simulink library "JT60SA_Magnetic_Control"  (R2019a)
settings: Solver=ode45  StartTime=0.0  StopTime=10.0  RelTol=1e-3  EnableMultiTasking=on
values from neighbouring files (symbols this model uses):
  Input_struct =     [SOF18d66_setup.mat]
  Ip0 = 5499999.99826    [SOF18d66_setup.mat]
  IVC_sat = 1000    [SOF18d66_setup.mat]
undefined symbols (not defined in the file or in its folder): iLow, Ip_PID, iUp, r_grid, R_grid, Rt, z_grid, Z_grid, Zt
libraries: simulink x2, cstblocks x2
settings Model: Creator=Adriano  LastModifiedBy=adria
settings DataIOCC: LimitDataPoints=on  SaveFormat=Array  ReturnWorkspaceOutputs=off
settings OptimizationCC: LifeSpan=inf
settings DebuggingCC: SFUnexpectedBacktrackingDiag=warning  SFNoUnconditionalDefaultTransitionDiag=warning  SFExecutionAtInitializationDiag=none  ArithmeticOperatorsInVariantConditions=warning
settings HardwareCC: ProdBitPerPointer=32  ProdBitPerSizeT=32  ProdBitPerPtrDiffT=32  ProdLargestAtomicFloat=None  ProdIntDivRoundTo=Undefined  ProdEndianess=Unspecified  ProdWordSize=32  ProdHWDeviceType=32-bit Generic
settings ModelReferenceCC: PropagateSignalLabelsOutOfModel=off
settings SFSimCC: SimUseLocalCustomCode=off
settings RTWCC: RTWUseLocalCustomCode=off
settings CodeAppCC: StateflowObjectComments=on
settings GRTTargetCC: TargetLangStandard=C89/C90 (ANSI)  GeneratePreprocessorConditionals=Disable all
settings ConfigComp: CovMetricSettings=dw  CovHtmlReporting=on  CovSaveCumulativeToWorkspaceVar=on  CovSaveSingleToWorkspaceVar=on  CovExternalEMLEnable=off

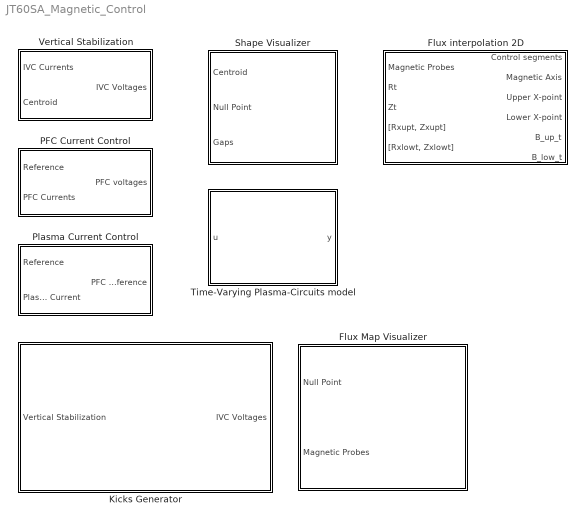
== system JT60SA_Magnetic_Control ==
  Flux Map Visualizer : Subsystem  InitFcn=|  StartFcn=% fig_grid= figure()
      | oldDir = pwd;
      | cd ./flux_grid_functions
      | [r_grid, z_grid, R_grid, Z_grid, F0, idxGrid] = initFluxGrid(Input_struct,y_np,y_type, mag, 0);
      | cd(oldDir);
      mask Display:
      | image(['.' filesep 'images' filesep 'Grid.jpg'])
      | port_label('input',1,'Null Point');
      | port_label('input',2, 'Mag Probes');
  Flux interpolation 2D : Subsystem  Description=|  InitFcn=|
      Description=|
      | This block allows to interpolate the flux map over a set of given control points.
      | 
      | The user must define Rt and Zt, which are 2 vectors of 20 elements which contain the coordinates
      | of the desired control points (only non-zero coordinate are used). Furthermore, the user must
      | define the desired position for the upper and lower X-points, [Rxupt, Zxupt] and [Rxlowt, Zxlowt]. 
      | The target points may be time varying.
      InitFcn=|
      | oldDir = pwd;
      | cd ./flux_grid_functions
      | [r_grid, z_grid, R_grid, Z_grid, F0, idxGrid] = initFluxGrid(Input_struct,y_np,y_type, mag, 0);
      | 
      | xpLow_guess = [Null0(1) -abs(Null0(2))];
      | [RBoxL, ZBoxL, irowL, icolL, maskL] = initXBox(xpLow_guess, R_grid, Z_grid);
      | iLow = [irowL; icolL];
      | 
      | xpUp_guess = [Null0(1) +abs(Null0(2))];
      | [RBoxU, ZBoxU, irowU, icolU, maskU] = initXBox(xpUp_guess, R_grid, Z_grid);
      | iUp = [irowU; icolU];
      | 
      | cd(oldDir);
  Kicks Generator : Subsystem  mask{freq_kicks=5, duty_cycle=50, perc_up=45}
      mask prompts: freq_kicks "Frequence [Hz]"; duty_cycle "Duty cycle"; perc_up "%up"
      mask Display:
      | image(['.' filesep 'images' filesep 'Kicks.png']);
      | port_label('input',1,'Vertical Stabilization');
      | port_label('output',1,'IVC Voltages');
  PFC Current Control : Subsystem  InitFcn=|
      | % PFC Current Control
      | Kpcurr = [5.7832    1.2410     0           0           0            0          0.8592   0            0            0
      |                1.2410    5.7862    1.2432    0           0            0          0           0            0            0
      |                0            1.2432    5.7865    1.2414   0            0          0           0            0            0
      |                0            0            1.2414    5.7845   0            0          0           0            0            0
      |                0            0            0            0           10.9807  2.7576  0           0            0.8679    2.0055
      |                0            0            0            0           2.7576    9.5196  1.2014   0            0            0
      |                0.8592    0            0            0           0            1.2014  6.6407   0            0            0
      |                0            0            0            1.1486   0            0          0           12.5627  2.1557    1.7044
      |                0            0            0            0           0            0          0           2.1557    7.4827    3.7590
      |                0            0            0            0           2.0055    0          0           1.7044    3.7590   14.2743]; % Decoupling Matrix
      mask help: PF Coils Current Controller
      mask init:
      | Kpcurr = [5.7832   1.2410        0        0         0       0  0.8592        0        0         0
      |           1.2410   5.7862   1.2432        0         0       0       0        0        0         0
      |                0   1.2432   5.7865   1.2414         0       0       0        0        0         0
      |                0        0   1.2414   5.7845         0       0       0        0        0         0
      |                0        0        0        0   10.9807  2.7576       0        0   0.8679    2.0055
      |                0        0        0        0    2.7576  9.5196  1.2014        0        0         0
      |           0.8592        0        0        0         0  1.2014  6.6407        0        0         0
      |                0        0        0   1.1486         0       0       0  12.5627   2.1557    1.7044
      |                0        0        0        0         0       0       0   2.1557   7.4827    3.7590
      |                0        0        0        0    2.0055       0       0   1.7044   3.7590   14.2743];
  Plasma Current Control : Subsystem  InitFcn=|  mask{Ip_Kp=1e-3, Ip_Ki=35*1e-3}
      | % Ip Control
      |  KIp= [-0.4984  -0.4327  -0.4393 -0.4969  -0.0241 ...
      |         -0.0268  -0.2920  -0.1886  -0.0465  -0.0151]'; % Transformer currents pattern
      mask prompts: Ip_Kp "Proportional gain"; Ip_Ki "Integral gain"
      mask help: Plasma Current Controller
      mask init:
      | KIp= [-0.4984  -0.4327  -0.4393 -0.4969  -0.0241 ...
      |       -0.0268  -0.2920  -0.1886  -0.0465 -0.0151]'; % Transformer currents pattern, normalized
  Shape Visualizer : Subsystem  StartFcn=|
      | plasmaShape = figure('Position',[800, 0, 450, 650]);
      | xlabel('R');
      | ylabel('Z');
      | 
      | %h = pdemesh(Input_struct.p,Input_struct.e,[]);
      | %set(h,'Color','black');
      | %axis([0, 6, -4.5, 4.5]);
      | %axis equal;
      | %hold on
      | 
      | %plasmaShape.UserData.plot = plot(zeros(nGaps,1), zeros(nGaps,1));
      mask help: Plasma Shape Visualizer
      mask Display:
      | image(['.' filesep 'images' filesep 'Shape.JPG']);
      | port_label('input',1,'Centroid');
      | port_label('input',2, 'Null Point');
      | port_label('input',3, 'Gaps');
  Time-Varying Plasma-Circuits model : Subsystem  InitFcn=|
      | if ~exist('equ_struct', 'var')
      |   try
      |       firstEquil = [pathName, fileName];
      |   catch
      |   end
      | 
      |   addpath(['.' filesep 'time-varying_model'])
      |   gen_equil_struct;
      | 
      | else
      |   warndlg('Equilibria structure already exists!');
      | end
      mask help: Time-Varying Plasma-Circuits linearized model.
      settings: DeleteFcn=clear equ_struct
      settings: CopyFcn=|
      | if ~exist('equ_struct', 'var')
      |   try
      |       firstEquil = [pathName, fileName];
      |   catch
      |   end
      | 
      |   addpath(['.' filesep 'time-varying_model'])
      |   gen_equil_struct;
      | else
      |   warndlg('Equilibria structure already exists!')
      | end
      mask Help:
      | This block contains a Time-Varying Plasma-Circuits model.
      | At the initialization, the user is asked to choose the equilibria to load
      | (the first one is the one currently loaded in the workspace). After this,
      | the user is asked to specify a time vector (one time istant for each model).
      | This block can be substituted to the blocks CREATE Model, Equilibrium
      | Inputs and Equilibrium Outputs under the Plasma-Circuits Linearized Model
      | mask (please note that the equilibrium inputs and outputs are already
      | taken into account, so the must not be added externally).
      | 
      | In the workspace, a structure named equ_struct will be available,
      | containing, among the other fields, the scenario currents for each of the
      | equilibria (these can be interpolated to build the current feedforward to
      | the model).
  Vertical Stabilization : Subsystem  InitFcn=|  mask{Zdot_Gain=-20/5.5e6, IVC_Gain=0.0076, VS_Gain=40}
      | % Vertical Stabilization
      | Zdot_Gain = 20;
      | IVC_Gain  = -0.0076;
      | VS_Gain   = -40;
      | derivativeFilter = tf([1, 0], [1/1000, 1]);
      mask prompts: Zdot_Gain "Velocity Gain/Ip"; IVC_Gain "Current Gain"; VS_Gain "Overall Gain"
      mask help: Vertical Stabilization Controller
      mask init:
      | % Zdot_Gain = 20/5.5e6;
      | % IVC_Gain  = -0.0076;
      | % VS_Gain   = -40;
      | 
      | derivativeFilter = tf([1, 0], [1/1000, 1]);

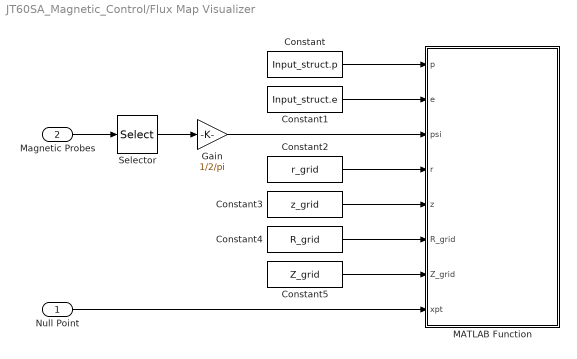
== system JT60SA_Magnetic_Control/Flux Map Visualizer ==
  Null Point : Inport
  Magnetic Probes : Inport  Port=2
  Constant : Constant  Value=Input_struct.p
  Constant1 : Constant  Value=Input_struct.e
  Constant2 : Constant  Value=r_grid
  Constant3 : Constant  Value=z_grid
  Constant4 : Constant  Value=R_grid
  Constant5 : Constant  Value=Z_grid
  Gain : Gain  Gain=1/2/pi
  MATLAB Function : MATLAB Function  TreatAsAtomicUnit=on  SystemSampleTime=5e-2
  Selector : Selector  InputPortWidth=nMag  IndexOptions=Index vector (dialog)  Indices=idxGrid  OutputSizes=1
  wires:
  Magnetic Probes/1 -> Selector/1
  Selector/1 -> Gain/1
  Constant/1 -> MATLAB Function/1(p)
  Constant1/1 -> MATLAB Function/2(e)
  Constant2/1 -> MATLAB Function/4(r)
  Constant3/1 -> MATLAB Function/5(z)
  Constant4/1 -> MATLAB Function/6(R_grid)
  Constant5/1 -> MATLAB Function/7(Z_grid)
  Null Point/1 -> MATLAB Function/8(xpt)
  Gain/1 -> MATLAB Function/3(psi)

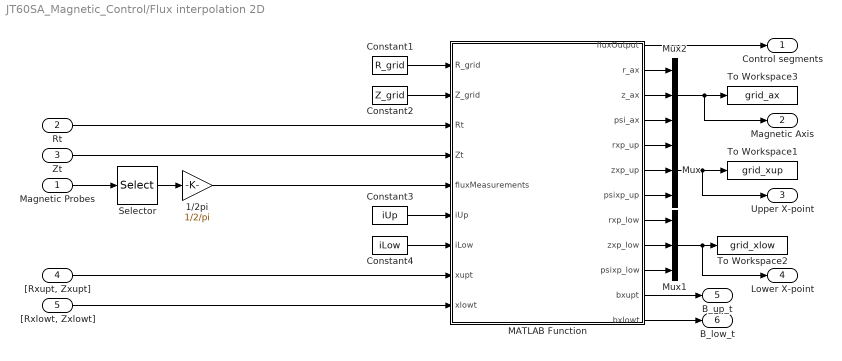
== system JT60SA_Magnetic_Control/Flux interpolation 2D ==
  Magnetic Probes : Inport
  Rt : Inport  Port=2
  Zt : Inport  Port=3
  "[Rxupt, Zxupt]" : Inport  Port=4
  "[Rxlowt, Zxlowt]" : Inport  Port=5
  1/2pi : Gain  Gain=1/2/pi
  Constant1 : Constant  Value=R_grid
  Constant2 : Constant  Value=Z_grid
  Constant3 : Constant  Value=iUp
  Constant4 : Constant  Value=iLow
  MATLAB Function : MATLAB Function  TreatAsAtomicUnit=on
  Mux : Mux  Inputs=3
  Mux1 : Mux  Inputs=3
  Mux2 : Mux  Inputs=3
  Selector : Selector  InputPortWidth=nMag  IndexOptions=Index vector (dialog)  Indices=idxGrid  OutputSizes=1
  To Workspace1 : ToWorkspace  VariableName=grid_xup  SaveFormat=Structure With Time  SampleTime=-1
  To Workspace2 : ToWorkspace  VariableName=grid_xlow  SaveFormat=Structure With Time  SampleTime=-1
  To Workspace3 : ToWorkspace  VariableName=grid_ax  SaveFormat=Structure With Time  SampleTime=-1
  Control segments : Outport
  Magnetic Axis : Outport  Port=2
  Upper X-point : Outport  Port=3
  Lower X-point : Outport  Port=4
  B_up_t : Outport  Port=5
  B_low_t : Outport  Port=6
  wires:
  Rt/1 -> MATLAB Function/3(Rt)
  Constant1/1 -> MATLAB Function/1(R_grid)
  Constant2/1 -> MATLAB Function/2(Z_grid)
  MATLAB Function/1(fluxOutput) -> Control segments/1
  Selector/1 -> 1/2pi/1
  Zt/1 -> MATLAB Function/4(Zt)
  Constant3/1 -> MATLAB Function/6(iUp)
  Constant4/1 -> MATLAB Function/7(iLow)
  MATLAB Function/5(rxp_up) -> Mux/1
  MATLAB Function/7(psixp_up) -> Mux/3
  MATLAB Function/6(zxp_up) -> Mux/2
  Mux/1 -> Upper X-point/1, To Workspace1/1
  MATLAB Function/8(rxp_low) -> Mux1/1
  MATLAB Function/9(zxp_low) -> Mux1/2
  MATLAB Function/10(psixp_low) -> Mux1/3
  Mux1/1 -> Lower X-point/1, To Workspace2/1
  MATLAB Function/2(r_ax) -> Mux2/1
  MATLAB Function/3(z_ax) -> Mux2/2
  MATLAB Function/4(psi_ax) -> Mux2/3
  Mux2/1 -> Magnetic Axis/1, To Workspace3/1
  MATLAB Function/11(bxupt) -> B_up_t/1
  "[Rxupt, Zxupt]"/1 -> MATLAB Function/8(xupt)
  "[Rxlowt, Zxlowt]"/1 -> MATLAB Function/9(xlowt)
  MATLAB Function/12(bxlowt) -> B_low_t/1
  Magnetic Probes/1 -> Selector/1
  1/2pi/1 -> MATLAB Function/5(fluxMeasurements)

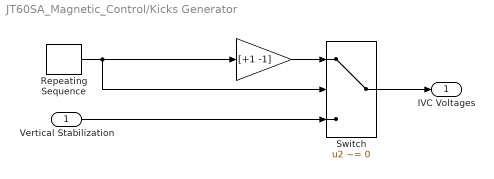
== system JT60SA_Magnetic_Control/Kicks Generator ==
  Vertical Stabilization : Inport
  "    " : Gain  Gain=[+1 -1]
  Repeating Sequence : simulink/Sources/Repeating Sequence  rep_seq_t="[0   (duty_cycle/100/freq_kicks)*(perc_up/100)+eps   (duty_cycle/100/freq_kicks)*(perc_up/100)+1.1*eps   duty_cycle/100/freq_kicks+1.2*eps  (duty_cycle/100/freq_kicks)+1.3*eps     1/freq_kicks+1.4*eps]"  rep_seq_y="[IVC_sat  IVC_sat   -IVC_sat  -IVC_sat  0  0]"
  Switch : Switch  Criteria=u2 ~= 0
  IVC Voltages : Outport
  wires:
  Switch/1 -> IVC Voltages/1
  "    "/1 -> Switch/1
  Repeating Sequence/1 -> "    "/1, Switch/2
  Vertical Stabilization/1 -> Switch/3

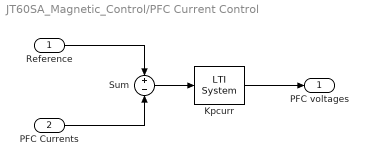
== system JT60SA_Magnetic_Control/PFC Current Control ==
  Reference : Inport
  PFC Currents : Inport  Port=2
  Kpcurr : cstblocks/LTI System  sys=Kpcurr  IC=[]
  Sum : Sum  Inputs=+-
  PFC voltages : Outport
  wires:
  Sum/1 -> Kpcurr/1
  PFC Currents/1 -> Sum/2
  Reference/1 -> Sum/1
  Kpcurr/1 -> PFC voltages/1

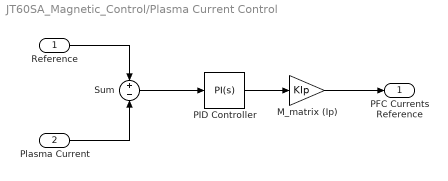
== system JT60SA_Magnetic_Control/Plasma Current Control ==
  Reference : Inport
  Plasma Current : Inport  Port=2
  M_matrix (Ip) : Gain  Gain=KIp
  PID Controller : simulink/Continuous/PID Controller  Controller=PI  Form=Parallel  TimeDomain=Continuous-time  SampleTime=-1  IntegratorMethod=Forward Euler  FilterMethod=Forward Euler  ControllerParametersSource=internal  P=Ip_Kp  I=Ip_Ki  D=Ip_PID.Kd  UseFilter=on  N=Ip_PID.Td  TunerSelectOption=Transfer Function Based (PID Tuner App)  InitialConditionSource=internal  InitialConditionForIntegrator=0  InitialConditionForFilter=0  DifferentiatorICPrevScaledInput=0  ExternalReset=none  TrackingMode=off  Kt=1  LimitOutput=off  UpperSaturationLimit=inf  LowerSaturationLimit=-inf  LinearizeAsGain=on  AntiWindupMode=none  Kb=1  POutMin=[]  POutMax=[]  IOutMin=[]  IOutMax=[]  DOutMin=[]  DOutMax=[]  NOutMin=[]  NOutMax=[]  SumOutMin=[]  SumOutMax=[]  SaturationOutMin=[]  SaturationOutMax=[]  PParamMin=[]  PParamMax=[]  IParamMin=[]  IParamMax=[]  DParamMin=[]  DParamMax=[]  NParamMin=[]  NParamMax=[]  KbParamMin=[]  KbParamMax=[]  KtParamMin=[]  KtParamMax=[]  KbOutMin=[]  KbOutMax=[]  KtOutMin=[]  KtOutMax=[]  IntegratorOutMin=[]  IntegratorOutMax=[]  FilterOutMin=[]  FilterOutMax=[]  SumI1OutMin=[]  SumI1OutMax=[]  SumI2OutMin=[]  SumI2OutMax=[]  SumI3OutMin=[]  SumI3OutMax=[]  SumI4OutMin=[]  SumI4OutMax=[]  SumDOutMin=[]  SumDOutMax=[]  DifferentiatorOutMin=[]  DifferentiatorOutMax=[]  FilterDiffOutCoefMin=[]  FilterDiffOutCoefMax=[]  ReciprocalOutMin=[]  ReciprocalOutMax=[]  SumDenOutMin=[]  SumDenOutMax=[]  SumNumOutMin=[]  SumNumOutMax=[]  DivideOutMin=[]  DivideOutMax=[]  IntegratorContinuousStateAttributes=''  IntegratorStateMustResolveToSignalObject=off  IntegratorRTWStateStorageClass=Auto  FilterContinuousStateAttributes=''  FilterStateMustResolveToSignalObject=off  FilterRTWStateStorageClass=Auto  ParallelPVariant=InternalParameters  IdealPVariant=Disabled  IVariant=InternalParameters  DVariant=Disabled  IntegratorVariant=Continuous  SatVariant=Disabled  AWVariant=Passthrough  PCopyVariant=Disabled  TRVariant=Disabled  FdbkBlocksVariant=Forward  IdealPFdbkVariant=Disabled  SatFdbkVariant=Disabled  DerivativeFilterVariant=Disabled  NVariant=Disabled  NCopyVariant=Disabled_SignalSpec  FilterICVariant=Disabled  IntegratorICVariant=InternalICs  ExternalResetVariant=Disabled  TRSumVariant=Passthrough  SumFdbkVariant=Disabled  SumVariant=Sum_PI
  Sum : Sum  Inputs=+-
  PFC Currents Reference : Outport
  wires:
  M_matrix (Ip)/1 -> PFC Currents Reference/1
  Sum/1 -> PID Controller/1
  PID Controller/1 -> M_matrix (Ip)/1
  Reference/1 -> Sum/1
  Plasma Current/1 -> Sum/2

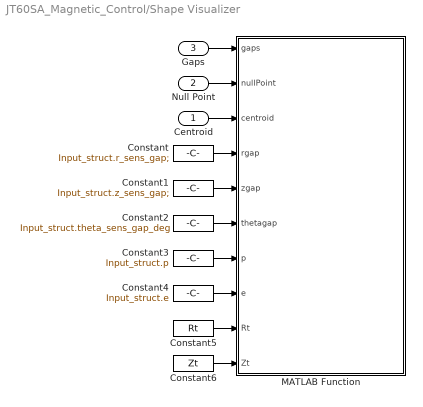
== system JT60SA_Magnetic_Control/Shape Visualizer ==
  Centroid : Inport  OutDataTypeStr=double  SampleTime=.05
  Null Point : Inport  Port=2  OutDataTypeStr=double  SampleTime=.05
  Gaps : Inport  Port=3  OutDataTypeStr=double  SampleTime=.05
  Constant : Constant  Value=Input_struct.r_sens_gap;
  Constant1 : Constant  Value=Input_struct.z_sens_gap;
  Constant2 : Constant  Value=Input_struct.theta_sens_gap_deg
  Constant3 : Constant  Value=Input_struct.p
  Constant4 : Constant  Value=Input_struct.e
  Constant5 : Constant  Value=Rt
  Constant6 : Constant  Value=Zt
  MATLAB Function : MATLAB Function  TreatAsAtomicUnit=on
  wires:
  Constant/1 -> MATLAB Function/4(rgap)
  Constant1/1 -> MATLAB Function/5(zgap)
  Constant2/1 -> MATLAB Function/6(thetagap)
  Gaps/1 -> MATLAB Function/1(gaps)
  Constant3/1 -> MATLAB Function/7(p)
  Constant4/1 -> MATLAB Function/8(e)
  Null Point/1 -> MATLAB Function/2(nullPoint)
  Centroid/1 -> MATLAB Function/3(centroid)
  Constant5/1 -> MATLAB Function/9(Rt)
  Constant6/1 -> MATLAB Function/10(Zt)

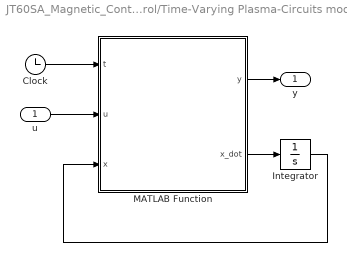
== system JT60SA_Magnetic_Control/Time-Varying Plasma-Circuits model ==
  u : Inport
  Clock : Clock
  Integrator : Integrator
  MATLAB Function : MATLAB Function  TreatAsAtomicUnit=on
  y : Outport
  wires:
  Clock/1 -> MATLAB Function/1(t)
  MATLAB Function/1(y) -> y/1
  u/1 -> MATLAB Function/2(u)
  MATLAB Function/2(x_dot) -> Integrator/1
  Integrator/1 -> MATLAB Function/3(x)

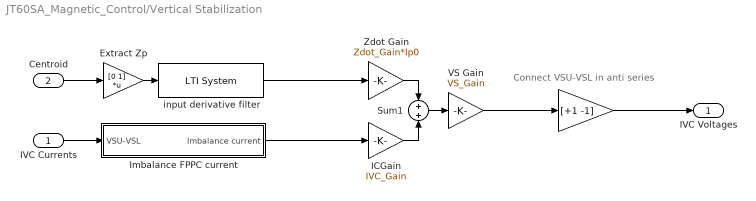
== system JT60SA_Magnetic_Control/Vertical Stabilization ==
  note: Connect VSU-VSL in anti series
  IVC Currents : Inport
  Centroid : Inport  Port=2
  "    " : Gain  Gain=[+1 -1]
  Extract Zp : Gain  Gain=[0 1]  Multiplication=Matrix(K*u)
  ICGain : Gain  Gain=IVC_Gain
  Imbalance FPPC current : Subsystem
  Sum1 : Sum  Inputs=+|+
  VS Gain : Gain  Gain=VS_Gain
  Zdot Gain : Gain  Gain=Zdot_Gain*Ip0
  input derivative filter : cstblocks/LTI System  sys=derivativeFilter  IC=[]
  IVC Voltages : Outport
  wires:
  IVC Currents/1 -> Imbalance FPPC current/1(VSU-VSL)
  input derivative filter/1 -> Zdot Gain/1
  Centroid/1 -> Extract Zp/1
  Sum1/1 -> VS Gain/1
  Zdot Gain/1 -> Sum1/1
  ICGain/1 -> Sum1/2
  "    "/1 -> IVC Voltages/1
  VS Gain/1 -> "    "/1
  Imbalance FPPC current/1(Imbalance current) -> ICGain/1
  Extract Zp/1 -> input derivative filter/1

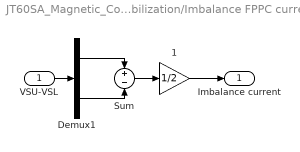
== system JT60SA_Magnetic_Control/Vertical Stabilization/Imbalance FPPC current ==
  VSU-VSL : Inport
  "    1" : Gain  Gain=1/2
  Demux1 : Demux  Outputs=2
  Sum : Sum  Inputs=+|-
  Imbalance current : Outport
  wires:
  VSU-VSL/1 -> Demux1/1
  "    1"/1 -> Imbalance current/1
  Demux1/2 -> Sum/2
  Sum/1 -> "    1"/1
  Demux1/1 -> Sum/1

== matlab function JT60SA_Magnetic_Control/Time-Varying Plasma-Circuits model/MATLAB Function ==
  data: equ_struct parameter; t input; u input size=equ_struct.sizeIn+2; y output size=equ_struct.sizeOut; x input; x_dot output size=equ_struct.sizeState
function [y,x_dot] = fcn(equ_struct,t,u,x)
%#codegen
coder.extrinsic('evalin');
coder.extrinsic('inv');
coder.extrinsic('horzcat');
% coder.extrinsic('mtimes');
% coder.extrinsic('mrdivide');
% coder.extrinsic('plus');
% coder.extrinsic('minus');

S = equ_struct;
y = zeros(equ_struct.sizeOut,1);
x_dot = zeros(equ_struct.sizeState,1);

L = zeros(size(S.L(:,:,1)));
R = zeros(size(S.R(:,:,1)));
C = zeros(size(S.C(:,:,1)));
D = zeros(size(S.D(:,:,1)));
F = zeros(size(S.F(:,:,1)));
E = zeros(size(S.E(:,:,1)));
LE = zeros(size(S.LE(:,:,1)));
u0 = zeros(size(S.u0(:,1)));
y0 = zeros(size(S.y0(:,1)));
W0 = zeros(size(S.W0(:,1)));
    
if S.time(1) >= t
    L = S.L(:,:,1);
    R = S.R(:,:,1);
    C = S.C(:,:,1);
    D = S.D(:,:,1);
    F = S.F(:,:,1);
    E = S.E(:,:,1);
    LE = S.LE(:,:,1);
    u0 = S.u0(:,1);
    y0 = S.y0(:,1);
    W0 = S.W0(:,1);
elseif (S.time(1) < t) && (S.time(end) > t)
    idx = find(S.time > t, 1);
    aa = (t-S.time(idx-1))/(S.time(idx)-S.time(idx-1));
    aa = aa(1);
    
    L = S.L(:,:,idx)*aa + S.L(:,:,idx-1)*(1-aa);
    R = S.R(:,:,idx)*aa + S.R(:,:,idx-1)*(1-aa);
    C = S.C(:,:,idx)*aa + S.C(:,:,idx-1)*(1-aa);
    D = S.D(:,:,idx)*aa + S.D(:,:,idx-1)*(1-aa);
    F = S.F(:,:,idx)*aa + S.F(:,:,idx-1)*(1-aa);
    % E = S.E(:,:,idx)*alpha + S.E(:,:,idx-1)*(1-alpha);
    LE = S.LE(:,:,idx)*aa + S.LE(:,:,idx-1)*(1-aa);
    u0 = S.u0(:,idx)*aa + S.u0(:,idx-1)*(1-aa);
    y0 = S.y0(:,idx)*aa + S.y0(:,idx-1)*(1-aa);
    W0 = S.W0(:,idx)*aa + S.W0(:,idx-1)*(1-aa);
    
    E = L\LE;
    
elseif S.time(end) <= t
    L = S.L(:,:,end);
    R = S.R(:,:,end);
    C = S.C(:,:,end);
    D = S.D(:,:,end);
    F = S.F(:,:,end);
    E = S.E(:,:,end);
    LE = S.LE(:,:,end);
    u0 = S.u0(:,end);
    y0 = S.y0(:,end);
    W0 = S.W0(:,end);
end

Linv = L\eye(size(L,1));
idxIn = S.idxIn;

%  Modify the model to take correctly into account the disturbances
idxIp = size(L,1);

idxI = setdiff(1:size(L,1), idxIp);
oldL = L;
oldC = C;


L(idxI,idxIp) = L(idxI,idxIp) + LE(idxI,:)*W0;

temp = LE(idxIp,:)*W0;
L(idxIp,idxIp) = L(idxIp,idxIp) + temp(1);

for i = 1 : size(C,1)
    temp = F(i,:)*W0;
    C(i,idxIp) = C(i,idxIp) + temp(1);
end
    
% Compute model matrices
ssA = -L\R;
ssB = Linv;
ssC = C;
ssD = D;

ssB = ssB(:, idxIn);

% State transformation to make the model compute the disturbances
% derivative
coder.extrinsic('mtimes');
coder.extrinsic('plus');

B2 = ssA*E;
ssB_new = [ssB, B2];

D2 = ssC*E + F;
ssD_new = [ssD, D2];

% Compute outputs
x_dot = ssA*x + ssB_new*(u-u0); % u0 already includes the disturbances!
y     = ssC*x + ssD_new*(u-u0) + y0;

== matlab function JT60SA_Magnetic_Control/Shape Visualizer/MATLAB Function ==
  data: gaps input; nullPoint input; centroid input; rgap input; zgap input; thetagap input; p input; e input; Rt input; Zt input
function fcn(gaps, nullPoint, centroid, rgap, zgap, thetagap, p, e, Rt, Zt)
coder.extrinsic('pdemesh');
coder.extrinsic('patch');

%#codegen
rx = nullPoint(1);
zx = nullPoint(2);

rp = centroid(1);
zp = centroid(2);

r = rgap+gaps.*cosd(thetagap);
z = zgap+gaps.*sind(thetagap);

rNew = r(~isnan(r)); % remove NaNs
zNew = z(~isnan(r));


%% Manipulate raw data

% strike points coordinates
if(zx < 0) % lower null
    idxStrike = find(zNew <= zx);
else       % upper null
    idxStrike = find(zNew >= zx);
end

rStrike = rNew(idxStrike); 
zStrike = zNew(idxStrike);

[~, idxLeft] = min(rStrike);
[~, idxRight] = max(rStrike);

% boundary points coordinates
idxBound = setdiff(1:length(rNew),idxStrike); 
rBound = rNew(idxBound);
zBound = zNew(idxBound);

rPlot = [rx; rBound];
zPlot = [zx; zBound];

% sort gaps
theta = atan2(zPlot-zp, rPlot-rp); 
% theta(theta<0) = theta(theta<0) + 2*pi;
[~, sortIdx] = sort(theta);
plotIdx = [sortIdx; sortIdx(1)];

%% Plot the plasma boundary
gcf;
xlabel('R')
ylabel('Z')

hold off
h = pdemesh(p,e,[]);
set(h,'Color','black');
% set(h, 'LineWidth',2);
axis([0, 6, -4.5, 4.5]), axis equal, hold on

patch(rPlot(plotIdx), zPlot(plotIdx),'m');
plot([rx, rStrike(idxLeft)], [zx, zStrike(idxLeft)], 'k');
plot([rx, rStrike(idxRight)], [zx, zStrike(idxRight)], 'k');
plot(rp,zp,'+k', 'LineWidth', 2);
plot(rx,zx,'xk', 'LineWidth', 2);


%% Plot the reference shape

if Rt~=0
    plot(Rt, Zt, '*r', 'LineWidth', 2);
end


% plot(r,z,'r');


% plasmaShape.UserData.plot.XData = r;
% plasmaShape.UserData.plot.YData = z;

% plasmaShape.userData.shapeHandle = line(r,z);
% plot(r,z,'b');

% plasmaShape.UserData.shapeHandle.XDataSource = 'r';
% plasmaShape.UserData.shapeHandle.YDataSource = 'z';
% refreshdata(plasmaShape);


% pdemesh(p,e,[]);
% axis([0, 6, -4.5, 4.5]);
% axis equal;
% hold on
% plot(r,z,'xb');


% 
% plasmaShape.UserData.shapeHandle.XData = r(idx)';
% plasmaShape.UserData.shapeHandle.YData = z(idx)';

== matlab function JT60SA_Magnetic_Control/Flux Map Visualizer/MATLAB Function ==
  data: p input; e input; psi input; r input; z input; R_grid input; Z_grid input; xpt input
function plotFluxMap(p,e,psi,r,z,R_grid,Z_grid,xpt)
%#codegen
coder.extrinsic('pdemesh');
coder.extrinsic('fit');
coder.extrinsic('feval');
coder.extrinsic('contour');

psib = xpt(3);

gcf
hold off
h = pdemesh(p,e,[]);
set(h,'Color','black');
axis([0, 6, -4.5, 4.5]), axis equal, hold on

sf = fit([r, z],psi,'linearinterp');      
FF = feval(sf,R_grid,Z_grid);
contour(R_grid,Z_grid,FF, 10);

[~,h] = contour(R_grid,Z_grid,FF, psib*[1 1]);
set(h, 'Color', 'k', 'LineWidth',1.2);

plot(xpt(1), xpt(2), 'ok');

== matlab function JT60SA_Magnetic_Control/Flux interpolation 2D/MATLAB Function ==
  data: R_grid input; fluxOutput output; r_ax output; z_ax output; psi_ax output; Z_grid input; Rt input; Zt input; fluxMeasurements input; iUp input; iLow input; rxp_up output; zxp_up output; psixp_up output; rxp_low output; zxp_low output; psixp_low output; xupt input; bxupt output; xlowt input; bxlowt output
function [fluxOutput, ...
          r_ax, z_ax, psi_ax, ...
          rxp_up, zxp_up, psixp_up, ...
          rxp_low, zxp_low, psixp_low, ...
          bxupt, bxlowt] = ...
          interpolateFluxes2D(R_grid,Z_grid, Rt,Zt, fluxMeasurements, iUp, iLow, xupt, xlowt)

fluxOutput = zeros(20, 1);

% Transform the output vector into a mesh
Nr = size(R_grid,2);
Nz = size(Z_grid,1);
F = zeros(Nr,Nz);
for i = 1 : Nr
    for j = 1 : Nz
        F(j,i) = fluxMeasurements((i-1)*Nr+j);
    end
end

% Compute the flux in the control points
for i = 1 : length(Rt)
    if Rt(i) == 0
        fluxOutput(i,1) = 0;
    else
        fluxOutput(i,1) = interp2(R_grid, Z_grid, F, Rt(i), Zt(i), 'spline');
    end
end

%%% Compute some interesting stuff from the flux map %%%%%%%%%%%%%%%%%%%%%%
%% Br Bz (not among the outputs for now)
dr = diff(R_grid(1,:));
dz = diff(Z_grid(:,1));
[FR,FZ] = gradient(F,dr(1),dz(1));
% From Grad-Shafranov eqn., we know that 
% Bz = (1/2*pi*r)*(dpsi/dr)   and    Br = -(1/2*pi*r)*(dpsi/dz)
Bz =  (1/2/pi)*(FR./R_grid);
Br = -(1/2/pi)*(FZ./R_grid);


%% Magnetic Axis
[ff,ir] = max(F);
[~, ic] = max(ff);
ir = min(ir(ic),100);
ic = min(ic, 100);

i_row = linspace(ir-2,ir+2,5); % box 5x5 (intorno al centro del plasma dovrebbe essere sempre ben definito)
i_col = linspace(ic-2,ic+2,5);

RBox = R_grid(i_row,i_col);
ZBox = Z_grid(i_row,i_col);
PsiBox = F(i_row,i_col);

Nr = size(RBox, 2);
Nz = size(ZBox, 1);

rr = reshape(RBox,[Nr*Nz, 1]);
zz = reshape(ZBox,[Nr*Nz, 1]);
ff = reshape(PsiBox,[Nr*Nz, 1]);

r_cc = RBox(1,(Nr+1)/2);
z_cc = ZBox((Nz+1)/2,1);
psi_cc = PsiBox((Nz+1)/2,(Nr+1)/2);

% Compute coefficients of the quadratic interpolation
dr = rr - r_cc;
dz = zz - z_cc;
dr2 = dr.^2;
dz2 = dz.^2;
drz = dr.*dz;
coeff = pinv([dr dz 0.5*dr2 drz 0.5*dz2])*(ff-psi_cc);

% Impose grad(poly) = 0
dXP = zeros(2,size(coeff,2));
dpsi_XP = zeros(1,size(coeff,2));
for i = 1 : size(coeff,2) % more than 1 iteration if more than 1 sensor box is considered
    h = [coeff(1,i) coeff(2,i)]';
    R = [coeff(3,i) coeff(4,i); coeff(4,i) coeff(5,i)];
    dXP(:,i) = -inv(R)*h;
    dpsi_XP(i) = h'*dXP(:,i)+0.5*dXP(:,i)'*R*dXP(:,i);
end

% Compute position, flux and field
r_ax   = r_cc + dXP(1,:); 
z_ax   = z_cc + dXP(2,:); 
psi_ax = psi_cc + dpsi_XP;
% br_ax  = interp2(R_grid, Z_grid, Br, r_ax, z_ax, 'cubic');
% bz_ax  = interp2(R_grid, Z_grid, Bz, r_ax, z_ax, 'cubic');


%% X point position, flux and field
% We need to find the point corresponding to zero flux gradient. The search
% could be restricted to some specific areas (see interpolation routines
% from Roberto and Antonio).

% define RBox, ZBox, PsiBox for upper and lower null

%% Upper x point 
i_row = iUp(1,:);
i_col = iUp(2,:);

RBox = R_grid(i_row,i_col);
ZBox = Z_grid(i_row,i_col);
PsiBox = F(i_row,i_col);

Nr = size(RBox, 2);
Nz = size(ZBox, 1);

rr = reshape(RBox,[Nr*Nz, 1]);
zz = reshape(ZBox,[Nr*Nz, 1]);
ff = reshape(PsiBox,[Nr*Nz, 1]);

r_cc = RBox(1,(Nr+1)/2);
z_cc = ZBox((Nz+1)/2,1);
psi_cc = PsiBox((Nz+1)/2,(Nr+1)/2);

% Compute coefficients of the quadratic interpolation
dr = rr - r_cc;
dz = zz- z_cc;
dr2 = dr.^2;
dz2 = dz.^2;
drz = dr.*dz;
coeff = pinv([dr dz 0.5*dr2 drz 0.5*dz2])*(ff-psi_cc);

% Impose grad(poly) = 0
dXP = zeros(2,size(coeff,2));
dpsi_XP = zeros(1,size(coeff,2));
for i = 1 : size(coeff,2) % more than 1 iteration if more than 1 sensor box is considered
    h = [coeff(1,i) coeff(2,i)]';
    R = [coeff(3,i) coeff(4,i); coeff(4,i) coeff(5,i)];
    dXP(:,i) = -inv(R)*h;
    dpsi_XP(i) = h'*dXP(:,i)+0.5*dXP(:,i)'*R*dXP(:,i);
end

% Compute position, flux and field
rxp_up   = r_cc + dXP(1,:);
zxp_up   = z_cc + dXP(2,:);
psixp_up = psi_cc + dpsi_XP;

brxp_up  = interp2(R_grid, Z_grid, Br, xupt(1), xupt(2), 'linear');
bzxp_up  = interp2(R_grid, Z_grid, Bz, xupt(1), xupt(2), 'linear');
bxupt = [brxp_up; bzxp_up];



%% Lower x point
i_row = iLow(1,:);
i_col = iLow(2,:);

RBox = R_grid(i_row,i_col);
ZBox = Z_grid(i_row,i_col);
PsiBox = F(i_row,i_col);

Nr = size(RBox, 2);
Nz = size(ZBox, 1);

rr = reshape(RBox,[Nr*Nz, 1]);
zz = reshape(ZBox,[Nr*Nz, 1]);
ff = reshape(PsiBox,[Nr*Nz, 1]);

r_cc = RBox(1,(Nr+1)/2);
z_cc = ZBox((Nz+1)/2,1);
psi_cc = PsiBox((Nz+1)/2,(Nr+1)/2);

% Compute coefficients of the quadratic interpolation
dr = rr - r_cc;
dz = zz- z_cc;
dr2 = dr.^2;
dz2 = dz.^2;
drz = dr.*dz;
coeff = pinv([dr dz 0.5*dr2 drz 0.5*dz2])*(ff-psi_cc);

% Impose grad(poly) = 0
dXP = zeros(2,size(coeff,2));
dpsi_XP = zeros(1,size(coeff,2));
for i=1:size(coeff,2) % more than 1 iteration if more than 1 sensor box is considered
    h = [coeff(1,i) coeff(2,i)]';
    R = [coeff(3,i) coeff(4,i); coeff(4,i) coeff(5,i)];
    dXP(:,i) = -inv(R)*h;
    dpsi_XP(i) = h'*dXP(:,i)+0.5*dXP(:,i)'*R*dXP(:,i);
end

% Compute position, flux and field
rxp_low   = r_cc + dXP(1,:);
zxp_low   = z_cc + dXP(2,:);
psixp_low = psi_cc + dpsi_XP;

brxp_low  = interp2(R_grid, Z_grid, Br, xlowt(1), xlowt(2), 'linear');
bzxp_low  = interp2(R_grid, Z_grid, Bz, xlowt(1), xlowt(2), 'linear');
bxlowt = [brxp_low; bzxp_low];




return















%% Gaps
% Vedi tra le routine, c'è già qualcosa(find gaps from flux map)


%% Magnetic field at the X-point target position
% rxt = xt(1);
% zxt = xt(2);
% brxt = interp2(R_grid, Z_grid, Br, rxt, zxt, 'cubic');
% bzxt = interp2(R_grid, Z_grid, Bz, rxt, zxt, 'cubic');
% bxt = [brxt; bzxt]; % just one target point for now!


%% dr_sep
% rr = 1.8 : 0.001 : 2.4;
% zz = zeros(size(rr));
% ff = interp2(R_grid, Z_grid, F, rr, zz)





end
